simulink model "fmu_v2_beta"  (R2021a)
settings: Solver=FixedStepAuto  StartTime=0.0  StopTime=10.0  FixedStep=framePeriod_s  RelTol=1e-3
undefined symbols (not defined in the file): framePeriod_s
settings Model: Creator=brian  LastModifiedBy=BrianTaylor
settings SolverCC: AlgebraicLoopSolver=TrustRegion
settings OptimizationCC: DefaultParameterBehavior=Inlined  GainParamInheritBuiltInType=on  UseFloatMulNetSlope=on  DefaultUnderspecifiedDataType=single  InlineInvariantSignals=on  PassReuseOutputArgsAs=Individual arguments  ZeroExternalMemoryAtStartup=off  ZeroInternalMemoryAtStartup=off  NoFixptDivByZeroProtection=on  EfficientFloat2IntCast=on  LifeSpan=1  OptimizeBlockOrder=speed  DifferentSizesBufferReuse=on  EfficientTunableParamExpr=on
settings DebuggingCC: ParameterTunabilityLossMsg=error  SFMachineParentedDataDiag=warning
settings HardwareCC: ProdBitPerPointer=32  ProdBitPerSizeT=32  ProdBitPerPtrDiffT=32  ProdLargestAtomicInteger=Long  ProdLargestAtomicFloat=Double  ProdWordSize=32  ProdLongLongMode=on  ProdHWDeviceType=NXP->Cortex-M4
settings ModelReferenceCC: ModelReferenceNumInstancesAllowed=Single
settings SFSimCC: SimParseCustomCode=off  MATLABDynamicMemAlloc=off
settings RTWCC: SystemTargetFile=ert.tlc  GenCodeOnly=on  TemplateMakefile=ert_default_tmf  RTWVerbose=off  BuildConfiguration=Faster Runs  TargetLang=C++
settings CodeAppCC: ForceParamTrailComments=on  IgnoreCustomStorageClasses=off  OperatorAnnotations=on  SimulinkDataObjDesc=on  SFDataObjDesc=on  CustomSymbolStrGlobalVar=rt$N$M  CustomSymbolStrType=$N$M  CustomSymbolStrFcn=$N$M$F  CustomSymbolStrMacro=$N$M  InsertBlockDesc=on
settings ERTTargetCC: TargetLangStandard=C++03 (ISO)  IncludeMdlTerminateFcn=off  CombineSignalStateStructs=on  SuppressErrorStatus=on  SupportAbsoluteTime=off  CodeInterfacePackaging=C++ class  SupportNonFinite=off  SupportComplex=off  ERTHeaderFileRootName=autocode$E  ERTSourceFileRootName=autocode$E  InlinedParameterPlacement=NonHierarchical  RootIOFormat=Structure reference  ERTCustomFileTemplate=example_file_process.tlc  ERTFilePackagingFormat=Compact  ArrayContainerType=std::array

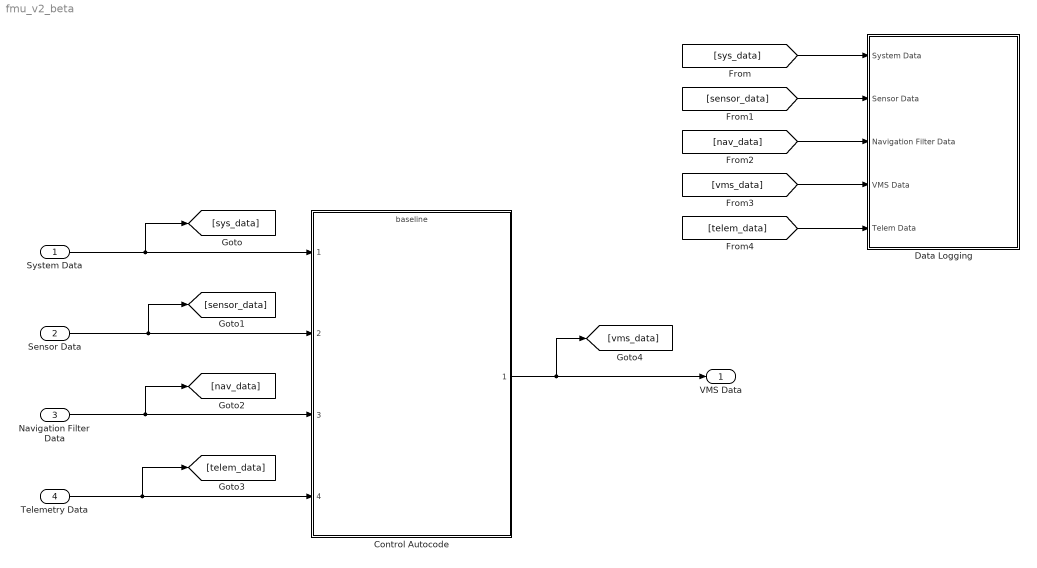
== system fmu_v2_beta ==
  System Data : Inport  OutDataTypeStr=Bus: SysData  SampleTime=framePeriod_s  BusOutputAsStruct=on
  Sensor Data : Inport  Port=2  OutDataTypeStr=Bus: SensorData  SampleTime=framePeriod_s  BusOutputAsStruct=on
  Navigation Filter Data : Inport  Port=3  OutDataTypeStr=Bus: NavData  SampleTime=framePeriod_s  BusOutputAsStruct=on
  Telemetry Data : Inport  Port=4  OutDataTypeStr=Bus: TelemData  SampleTime=framePeriod_s  BusOutputAsStruct=on
  Control Autocode : ModelReference  ModelNameDialog=baseline.slx  SimulationMode=Normal  ModelReferenceVersion=2.0
  Data Logging : Subsystem
  VMS Data : Outport  OutDataTypeStr=Bus: VmsData  SampleTime=framePeriod_s  BusOutputAsStruct=on
  wires:
  System Data/1 -> [sys_data], Control Autocode/1
  Sensor Data/1 -> [sensor_data], Control Autocode/2
  Navigation Filter Data/1 -> [nav_data], Control Autocode/3
  Telemetry Data/1 -> [telem_data], Control Autocode/4
  Control Autocode/1 -> [vms_data], VMS Data/1
  [telem_data] -> Data Logging/5(Telem Data)
  [vms_data] -> Data Logging/4(VMS Data)
  [sys_data] -> Data Logging/1(System Data)
  [nav_data] -> Data Logging/3(Navigation Filter Data)
  [sensor_data] -> Data Logging/2(Sensor Data)

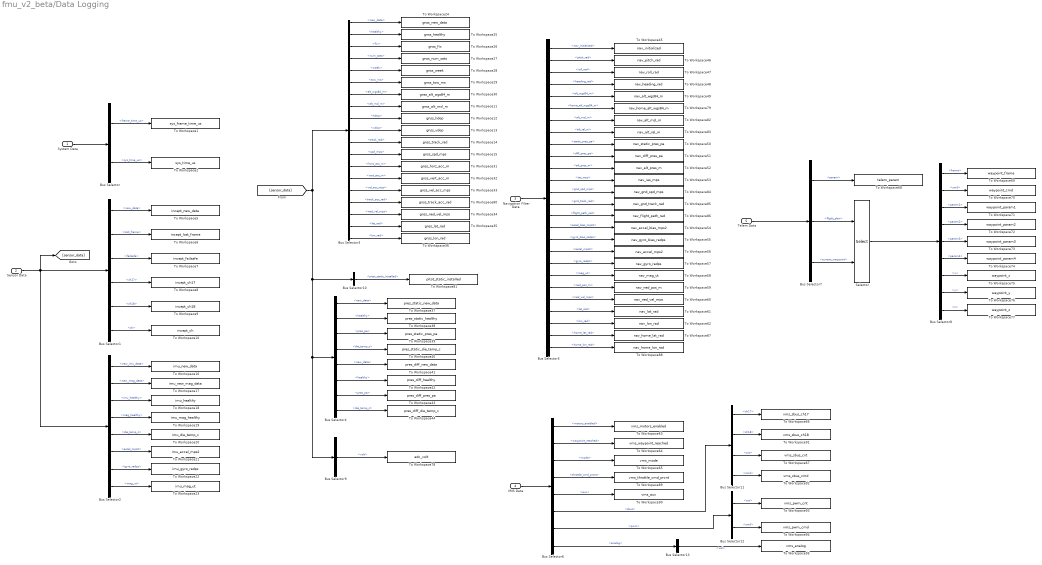
== system fmu_v2_beta/Data Logging ==
  System Data : Inport
  Sensor Data : Inport  Port=2
  Navigation Filter Data : Inport  Port=3
  VMS Data : Inport  Port=4
  Telem Data : Inport  Port=5
  Bus Selector : BusSelector  OutputSignals=frame_time_us,sys_time_us
  Bus Selector1 : BusSelector  OutputSignals=inceptor.new_data,inceptor.lost_frame,inceptor.failsafe,inceptor.ch17,inceptor.ch18,inceptor.ch
  Bus Selector10 : BusSelector  OutputSignals=pitot_static_installed
  Bus Selector11 : BusSelector  OutputSignals=ch17,ch18,cnt,cmd
  Bus Selector12 : BusSelector  OutputSignals=cnt,cmd
  Bus Selector13 : BusSelector  OutputSignals=val
  Bus Selector2 : BusSelector  OutputSignals=imu.new_imu_data,imu.new_mag_data,imu.imu_healthy,imu.mag_healthy,imu.die_temp_c,imu.accel_mps2,imu.gyro_radps,imu.mag_ut
  Bus Selector3 : BusSelector  OutputSignals=gnss.new_data,gnss.healthy,gnss.fix,gnss.num_sats,gnss.week,gnss.tow_ms,gnss.alt_wgs84_m,gnss.alt_msl_m,gnss.hdop,gnss.vdop,gnss.track_rad,gnss.spd_mps,gnss.horz_acc_m,gnss.vert_acc_m,gnss.vel_acc_mps,gnss.track_acc_rad,gnss.ned_vel_mps,gnss.lat_rad,gnss.lon_rad
  Bus Selector4 : BusSelector  OutputSignals=static_pres.new_data,static_pres.healthy,static_pres.pres_pa,static_pres.die_temp_c,diff_pres.new_data,diff_pres.healthy,diff_pres.pres_pa,diff_pres.die_temp_c
  Bus Selector5 : BusSelector  OutputSignals=nav_initialized,pitch_rad,roll_rad,heading_rad,alt_wgs84_m,home_alt_wgs84_m,alt_msl_m,alt_rel_m,static_pres_pa,diff_pres_pa,alt_pres_m,ias_mps,gnd_spd_mps,gnd_track_rad,flight_path_rad,accel_bias_mps2,gyro_bias_radps,accel_mps2,gyro_radps,mag_ut,ned_pos_m,ned_vel_mps,lat_rad,lon_rad,home_lat_rad,home_lon_rad
  Bus Selector6 : BusSelector  OutputSignals=motors_enabled,waypoint_reached,mode,throttle_cmd_prcnt,aux,sbus,pwm,analog
  Bus Selector7 : BusSelector  OutputSignals=param,flight_plan,current_waypoint
  Bus Selector8 : BusSelector  OutputSignals=frame,cmd,param1,param2,param3,param4,x,y,z
  Bus Selector9 : BusSelector  OutputSignals=adc.volt
  Selector : Selector  IndexMode=Zero-based  InputPortWidth=500  IndexOptions=Index vector (port)  Indices=[1 3]  OutputSizes=1
  To Workspace1 : ToWorkspace  VariableName=sys_frame_time_us  SampleTime=-1
  To Workspace10 : ToWorkspace  VariableName=incept_ch  SampleTime=-1
  To Workspace11 : ToWorkspace  VariableName=gnss_alt_msl_m  SampleTime=-1
  To Workspace12 : ToWorkspace  VariableName=gnss_hdop  SampleTime=-1
  To Workspace13 : ToWorkspace  VariableName=gnss_vdop  SampleTime=-1
  To Workspace14 : ToWorkspace  VariableName=gnss_track_rad  SampleTime=-1
  To Workspace15 : ToWorkspace  VariableName=gnss_spd_mps  SampleTime=-1
  To Workspace16 : ToWorkspace  VariableName=imu_new_data  SampleTime=-1
  To Workspace17 : ToWorkspace  VariableName=imu_new_mag_data  SampleTime=-1
  To Workspace18 : ToWorkspace  VariableName=imu_healthy  SampleTime=-1
  To Workspace19 : ToWorkspace  VariableName=imu_mag_healthy  SampleTime=-1
  To Workspace2 : ToWorkspace  VariableName=sys_time_us  SampleTime=-1
  To Workspace20 : ToWorkspace  VariableName=imu_die_temp_c  SampleTime=-1
  To Workspace21 : ToWorkspace  VariableName=imu_accel_mps2  SampleTime=-1
  To Workspace22 : ToWorkspace  VariableName=imu_gyro_radps  SampleTime=-1
  To Workspace23 : ToWorkspace  VariableName=imu_mag_ut  SampleTime=-1
  To Workspace24 : ToWorkspace  VariableName=gnss_new_data  SampleTime=-1
  To Workspace25 : ToWorkspace  VariableName=gnss_healthy  SampleTime=-1
  To Workspace26 : ToWorkspace  VariableName=gnss_fix  SampleTime=-1
  To Workspace27 : ToWorkspace  VariableName=gnss_num_sats  SampleTime=-1
  To Workspace28 : ToWorkspace  VariableName=gnss_week  SampleTime=-1
  To Workspace29 : ToWorkspace  VariableName=gnss_tow_ms  SampleTime=-1
  To Workspace30 : ToWorkspace  VariableName=gnss_alt_wgs84_m  SampleTime=-1
  To Workspace31 : ToWorkspace  VariableName=gnss_horz_acc_m  SampleTime=-1
  To Workspace32 : ToWorkspace  VariableName=gnss_vert_acc_m  SampleTime=-1
  To Workspace33 : ToWorkspace  VariableName=gnss_vel_acc_mps  SampleTime=-1
  To Workspace34 : ToWorkspace  VariableName=gnss_ned_vel_mps  SampleTime=-1
  To Workspace35 : ToWorkspace  VariableName=gnss_lat_rad  SampleTime=-1
  To Workspace36 : ToWorkspace  VariableName=gnss_lon_rad  SampleTime=-1
  To Workspace37 : ToWorkspace  VariableName=pres_static_new_data  SampleTime=-1
  To Workspace38 : ToWorkspace  VariableName=pres_static_healthy  SampleTime=-1
  To Workspace39 : ToWorkspace  VariableName=pres_static_pres_pa  SampleTime=-1
  To Workspace40 : ToWorkspace  VariableName=pres_static_die_temp_c  SampleTime=-1
  To Workspace41 : ToWorkspace  VariableName=pres_diff_new_data  SampleTime=-1
  To Workspace42 : ToWorkspace  VariableName=pres_diff_healthy  SampleTime=-1
  To Workspace43 : ToWorkspace  VariableName=pres_diff_pres_pa  SampleTime=-1
  To Workspace44 : ToWorkspace  VariableName=pres_diff_die_temp_c  SampleTime=-1
  To Workspace45 : ToWorkspace  VariableName=nav_initialized  SampleTime=-1
  To Workspace46 : ToWorkspace  VariableName=nav_pitch_rad  SampleTime=-1
  To Workspace47 : ToWorkspace  VariableName=nav_roll_rad  SampleTime=-1
  To Workspace48 : ToWorkspace  VariableName=nav_heading_rad  SampleTime=-1
  To Workspace49 : ToWorkspace  VariableName=nav_alt_wgs84_m  SampleTime=-1
  To Workspace5 : ToWorkspace  VariableName=incept_new_data  SampleTime=-1
  To Workspace50 : ToWorkspace  VariableName=nav_static_pres_pa  SampleTime=-1
  To Workspace51 : ToWorkspace  VariableName=nav_diff_pres_pa  SampleTime=-1
  To Workspace52 : ToWorkspace  VariableName=nav_alt_pres_m  SampleTime=-1
  To Workspace53 : ToWorkspace  VariableName=nav_ias_mps  SampleTime=-1
  To Workspace54 : ToWorkspace  VariableName=nav_accel_bias_mps2  SampleTime=-1
  To Workspace55 : ToWorkspace  VariableName=nav_gyro_bias_radps  SampleTime=-1
  To Workspace56 : ToWorkspace  VariableName=nav_accel_mps2  SampleTime=-1
  To Workspace57 : ToWorkspace  VariableName=nav_gyro_radps  SampleTime=-1
  To Workspace58 : ToWorkspace  VariableName=nav_mag_ut  SampleTime=-1
  To Workspace59 : ToWorkspace  VariableName=nav_ned_pos_m  SampleTime=-1
  To Workspace6 : ToWorkspace  VariableName=incept_lost_frame  SampleTime=-1
  To Workspace60 : ToWorkspace  VariableName=nav_ned_vel_mps  SampleTime=-1
  To Workspace61 : ToWorkspace  VariableName=nav_lat_rad  SampleTime=-1
  To Workspace62 : ToWorkspace  VariableName=nav_lon_rad  SampleTime=-1
  To Workspace63 : ToWorkspace  VariableName=vms_motors_enabled  SampleTime=-1
  To Workspace64 : ToWorkspace  VariableName=vms_waypoint_reached  SampleTime=-1
  To Workspace65 : ToWorkspace  VariableName=vms_mode  SampleTime=-1
  To Workspace66 : ToWorkspace  VariableName=vms_sbus_ch17  SampleTime=-1
  To Workspace67 : ToWorkspace  VariableName=vms_sbus_cnt  SampleTime=-1
  To Workspace68 : ToWorkspace  VariableName=telem_param  SampleTime=-1
  To Workspace69 : ToWorkspace  VariableName=waypoint_frame  SampleTime=-1
  To Workspace7 : ToWorkspace  VariableName=incept_failsafe  SampleTime=-1
  To Workspace70 : ToWorkspace  VariableName=waypoint_cmd  SampleTime=-1
  To Workspace71 : ToWorkspace  VariableName=waypoint_param1  SampleTime=-1
  To Workspace72 : ToWorkspace  VariableName=waypoint_param2  SampleTime=-1
  To Workspace73 : ToWorkspace  VariableName=waypoint_param3  SampleTime=-1
  To Workspace74 : ToWorkspace  VariableName=waypoint_param4  SampleTime=-1
  To Workspace75 : ToWorkspace  VariableName=waypoint_x  SampleTime=-1
  To Workspace76 : ToWorkspace  VariableName=waypoint_y  SampleTime=-1
  To Workspace77 : ToWorkspace  VariableName=waypoint_z  SampleTime=-1
  To Workspace78 : ToWorkspace  VariableName=adc_volt  SampleTime=-1
  To Workspace79 : ToWorkspace  VariableName=nav_home_alt_wgs84_m  SampleTime=-1
  To Workspace8 : ToWorkspace  VariableName=incept_ch17  SampleTime=-1
  To Workspace80 : ToWorkspace  VariableName=gnss_track_acc_rad  SampleTime=-1
  To Workspace81 : ToWorkspace  VariableName=pitot_static_installed  SampleTime=-1
  To Workspace82 : ToWorkspace  VariableName=nav_alt_msl_m  SampleTime=-1
  To Workspace83 : ToWorkspace  VariableName=nav_alt_rel_m  SampleTime=-1
  To Workspace84 : ToWorkspace  VariableName=nav_gnd_spd_mps  SampleTime=-1
  To Workspace85 : ToWorkspace  VariableName=nav_gnd_track_rad  SampleTime=-1
  To Workspace86 : ToWorkspace  VariableName=nav_flight_path_rad  SampleTime=-1
  To Workspace87 : ToWorkspace  VariableName=nav_home_lat_rad  SampleTime=-1
  To Workspace88 : ToWorkspace  VariableName=nav_home_lon_rad  SampleTime=-1
  To Workspace89 : ToWorkspace  VariableName=vms_throttle_cmd_prcnt  SampleTime=-1
  To Workspace9 : ToWorkspace  VariableName=incept_ch18  SampleTime=-1
  To Workspace90 : ToWorkspace  VariableName=vms_aux  SampleTime=-1
  To Workspace91 : ToWorkspace  VariableName=vms_sbus_ch18  SampleTime=-1
  To Workspace92 : ToWorkspace  VariableName=vms_sbus_cmd  SampleTime=-1
  To Workspace93 : ToWorkspace  VariableName=vms_pwm_cnt  SampleTime=-1
  To Workspace94 : ToWorkspace  VariableName=vms_pwm_cmd  SampleTime=-1
  To Workspace95 : ToWorkspace  VariableName=vms_analog  SampleTime=-1
  wires:
  System Data/1 -> Bus Selector/1
  Bus Selector/1 -> To Workspace1/1  "<frame_time_us>"
  Bus Selector/2 -> To Workspace2/1  "<sys_time_us>"
  Sensor Data/1 -> Bus Selector1/1, Bus Selector2/1, [sensor_data]
  Bus Selector2/1 -> To Workspace16/1  "<new_imu_data>"
  Bus Selector2/2 -> To Workspace17/1  "<new_mag_data>"
  Bus Selector2/3 -> To Workspace18/1  "<imu_healthy>"
  Bus Selector2/4 -> To Workspace19/1  "<mag_healthy>"
  Bus Selector2/5 -> To Workspace20/1  "<die_temp_c>"
  Bus Selector2/6 -> To Workspace21/1  "<accel_mps2>"
  Bus Selector2/7 -> To Workspace22/1  "<gyro_radps>"
  Bus Selector2/8 -> To Workspace23/1  "<mag_ut>"
  [sensor_data] -> Bus Selector10/1, Bus Selector9/1, Bus Selector4/1, Bus Selector3/1
  Bus Selector3/1 -> To Workspace24/1  "<new_data>"
  Bus Selector3/2 -> To Workspace25/1  "<healthy>"
  Bus Selector3/3 -> To Workspace26/1  "<fix>"
  Bus Selector3/4 -> To Workspace27/1  "<num_sats>"
  Bus Selector3/5 -> To Workspace28/1  "<week>"
  Bus Selector3/6 -> To Workspace29/1  "<tow_ms>"
  Bus Selector3/7 -> To Workspace30/1  "<alt_wgs84_m>"
  Bus Selector3/13 -> To Workspace31/1  "<horz_acc_m>"
  Bus Selector3/14 -> To Workspace32/1  "<vert_acc_m>"
  Bus Selector3/15 -> To Workspace33/1  "<vel_acc_mps>"
  Bus Selector3/17 -> To Workspace34/1  "<ned_vel_mps>"
  Bus Selector3/18 -> To Workspace35/1  "<lat_rad>"
  Bus Selector3/19 -> To Workspace36/1  "<lon_rad>"
  Bus Selector4/1 -> To Workspace37/1  "<new_data>"
  Bus Selector4/2 -> To Workspace38/1  "<healthy>"
  Bus Selector4/3 -> To Workspace39/1  "<pres_pa>"
  Bus Selector4/4 -> To Workspace40/1  "<die_temp_c>"
  Bus Selector4/5 -> To Workspace41/1  "<new_data>"
  Bus Selector4/6 -> To Workspace42/1  "<healthy>"
  Bus Selector4/7 -> To Workspace43/1  "<pres_pa>"
  Bus Selector4/8 -> To Workspace44/1  "<die_temp_c>"
  Navigation Filter Data/1 -> Bus Selector5/1
  Bus Selector5/1 -> To Workspace45/1  "<nav_initialized>"
  Bus Selector5/2 -> To Workspace46/1  "<pitch_rad>"
  Bus Selector5/3 -> To Workspace47/1  "<roll_rad>"
  Bus Selector5/4 -> To Workspace48/1  "<heading_rad>"
  Bus Selector5/5 -> To Workspace49/1  "<alt_wgs84_m>"
  Bus Selector5/9 -> To Workspace50/1  "<static_pres_pa>"
  Bus Selector5/10 -> To Workspace51/1  "<diff_pres_pa>"
  Bus Selector5/11 -> To Workspace52/1  "<alt_pres_m>"
  Bus Selector5/12 -> To Workspace53/1  "<ias_mps>"
  Bus Selector5/16 -> To Workspace54/1  "<accel_bias_mps2>"
  Bus Selector5/17 -> To Workspace55/1  "<gyro_bias_radps>"
  Bus Selector5/18 -> To Workspace56/1  "<accel_mps2>"
  Bus Selector5/19 -> To Workspace57/1  "<gyro_radps>"
  Bus Selector5/20 -> To Workspace58/1  "<mag_ut>"
  Bus Selector5/21 -> To Workspace59/1  "<ned_pos_m>"
  Bus Selector5/22 -> To Workspace60/1  "<ned_vel_mps>"
  Bus Selector5/23 -> To Workspace61/1  "<lat_rad>"
  Bus Selector5/24 -> To Workspace62/1  "<lon_rad>"
  VMS Data/1 -> Bus Selector6/1
  Telem Data/1 -> Bus Selector7/1
  Bus Selector7/1 -> To Workspace68/1  "<param>"
  Bus Selector7/2 -> Selector/1  "<flight_plan>"
  Bus Selector7/3 -> Selector/2  "<current_waypoint>"
  Selector/1 -> Bus Selector8/1
  Bus Selector8/1 -> To Workspace69/1  "<frame>"
  Bus Selector8/2 -> To Workspace70/1  "<cmd>"
  Bus Selector8/3 -> To Workspace71/1  "<param1>"
  Bus Selector8/4 -> To Workspace72/1  "<param2>"
  Bus Selector8/5 -> To Workspace73/1  "<param3>"
  Bus Selector8/6 -> To Workspace74/1  "<param4>"
  Bus Selector8/7 -> To Workspace75/1  "<x>"
  Bus Selector8/8 -> To Workspace76/1  "<y>"
  Bus Selector8/9 -> To Workspace77/1  "<z>"
  Bus Selector9/1 -> To Workspace78/1  "<volt>"
  Bus Selector1/1 -> To Workspace5/1  "<new_data>"
  Bus Selector1/2 -> To Workspace6/1  "<lost_frame>"
  Bus Selector1/3 -> To Workspace7/1  "<failsafe>"
  Bus Selector1/4 -> To Workspace8/1  "<ch17>"
  Bus Selector1/5 -> To Workspace9/1  "<ch18>"
  Bus Selector1/6 -> To Workspace10/1  "<ch>"
  Bus Selector3/8 -> To Workspace11/1  "<alt_msl_m>"
  Bus Selector3/9 -> To Workspace12/1  "<hdop>"
  Bus Selector3/10 -> To Workspace13/1  "<vdop>"
  Bus Selector3/11 -> To Workspace14/1  "<track_rad>"
  Bus Selector3/12 -> To Workspace15/1  "<spd_mps>"
  Bus Selector3/16 -> To Workspace80/1  "<track_acc_rad>"
  Bus Selector10/1 -> To Workspace81/1  "<pitot_static_installed>"
  Bus Selector5/6 -> To Workspace79/1  "<home_alt_wgs84_m>"
  Bus Selector5/7 -> To Workspace82/1  "<alt_msl_m>"
  Bus Selector5/8 -> To Workspace83/1  "<alt_rel_m>"
  Bus Selector5/13 -> To Workspace84/1  "<gnd_spd_mps>"
  Bus Selector5/14 -> To Workspace85/1  "<gnd_track_rad>"
  Bus Selector5/15 -> To Workspace86/1  "<flight_path_rad>"
  Bus Selector5/25 -> To Workspace87/1  "<home_lat_rad>"
  Bus Selector5/26 -> To Workspace88/1  "<home_lon_rad>"
  Bus Selector6/1 -> To Workspace63/1  "<motors_enabled>"
  Bus Selector6/2 -> To Workspace64/1  "<waypoint_reached>"
  Bus Selector6/3 -> To Workspace65/1  "<mode>"
  Bus Selector6/4 -> To Workspace89/1  "<throttle_cmd_prcnt>"
  Bus Selector6/5 -> To Workspace90/1  "<aux>"
  Bus Selector6/6 -> Bus Selector11/1  "<sbus>"
  Bus Selector11/1 -> To Workspace66/1  "<ch17>"
  Bus Selector11/2 -> To Workspace91/1  "<ch18>"
  Bus Selector11/3 -> To Workspace67/1  "<cnt>"
  Bus Selector11/4 -> To Workspace92/1  "<cmd>"
  Bus Selector6/7 -> Bus Selector12/1  "<pwm>"
  Bus Selector12/1 -> To Workspace93/1  "<cnt>"
  Bus Selector12/2 -> To Workspace94/1  "<cmd>"
  Bus Selector6/8 -> Bus Selector13/1  "<analog>"
  Bus Selector13/1 -> To Workspace95/1  "<val>"
